simulink model "lego_selfbalance_students"  (R2014a)
settings: Solver=ode3  SolverMode=SingleTasking  StartTime=0.0  StopTime=inf  RelTol=1e-3
values from neighbouring files (symbols this model uses):
  A1 = [ ... (first row only)    [lego_selfbalance_parameters.m]
  A2 = [ ... (first row only)    [lego_selfbalance_parameters.m]
  a_b = 0.8    [lego_selfbalance_parameters.m]
  a_d = 0.8    [lego_selfbalance_parameters.m]
  a_gc = 0.8    [lego_selfbalance_parameters.m]
  a_gd = 0.999    [lego_selfbalance_parameters.m]
  a_r = 0.996    [lego_selfbalance_parameters.m]
  B1 = [ ... (first row only)    [lego_selfbalance_parameters.m]
  B2 = [ ... (first row only)    [lego_selfbalance_parameters.m]
  BATTERY = 8000    [lego_selfbalance_parameters.m]
  C1 = eye(4)    [lego_selfbalance_parameters.m]
  C2 = eye(2)    [lego_selfbalance_parameters.m]
  D = 0.04    [lego_selfbalance_parameters.m]
  D1 = zeros(4, 2)    [lego_selfbalance_parameters.m]
  D2 = zeros(2)    [lego_selfbalance_parameters.m]
  GYRO0 = 600    [lego_selfbalance_parameters.m]
  k_sync = 0.35    [lego_selfbalance_parameters.m]
  pwm_gain = 1    [lego_selfbalance_parameters.m]
  pwm_offset = 0    [lego_selfbalance_parameters.m]
  R = 0.04    [lego_selfbalance_parameters.m]
  START_POS = [100, 100]    [lego_selfbalance_parameters.m]
  time_start = 4000    [lego_selfbalance_parameters.m]
  TS = 0.001    [lego_selfbalance_parameters.m]
  ts1 = 0.004    [lego_selfbalance_parameters.m]
  W = 0.14    [lego_selfbalance_parameters.m]
  X1IV = [ ... (first row only)    [lego_selfbalance_parameters.m]
  X2IV = [ ... (first row only)    [lego_selfbalance_parameters.m]
undefined symbols (not defined in the file or in its folder): DiscIntNeverNeededParam
libraries: legonxtlib x8, simulink x3
PreSaveFcn:
  | set_param(gcs, 'Location',[35 56 895 605])
settings Model: FPTRunName=Active  SimulationMode=external  ExtModeTrigDuration=2  Creator=The MathWorks Inc.  LastModifiedBy=Dan
settings DataIOCC: SignalLoggingSaveFormat=ModelDataLogs
settings OptimizationCC: ExpressionDepthLimit=2147483647  OptimizeModelRefInitCode=on  LifeSpan=Inf
settings DebuggingCC: UnderspecifiedInitializationDetection=Classic  SolverPrmCheckMsg=none  FcnCallInpInsideContextMsg=EnableAllAsWarning  StateNameClashWarn=warning
settings HardwareCC: ProdLargestAtomicInteger=Long  ProdLargestAtomicFloat=Float  ProdEndianess=LittleEndian  ProdHWDeviceType=ARM Compatible->ARM 7
settings RTWCC: SystemTargetFile=realtime.tlc  GenerateMakefile=off  TemplateMakefile=realtime.tmf  Description=Run on Target Hardware  RTWVerbose=off  ProcessScript=realtime_make_rtw_hook
settings CodeAppCC: CustomSymbolStrType=$N$R$M  InternalIdentifier=Classic
settings STFCustomTargetCC: TargetLibSuffix=.a  GenerateSampleERTMain=on  ConcurrentExecutionCompliant=off  GeneratePreprocessorConditionals=Use local settings  ERTCustomFileBanners=on  SupportNonInlinedSFcns=off  SupportVariableSizeSignals=on  MATLABClassNameForMDSCustomization=Simulink.SoftwareTarget.ERTCustomization  GRTInterface=off  SystemTargetFile=realtime.tlc
settings ERTTargetCC: CombineOutputUpdateFcns=off  SupportContinuousTime=on  SupportVariableSizeSignals=on  ExtMode=on  ExtModeTransport=2  ExtModeMexArgs=0 13 9600 30  ERTSrcFileBannerTemplate=realtime_code_template.cgt  ERTHdrFileBannerTemplate=realtime_code_template.cgt  ERTDataSrcFileTemplate=realtime_code_template.cgt  ERTDataHdrFileTemplate=realtime_code_template.cgt  ERTCustomFileTemplate=realtime_file_process.tlc

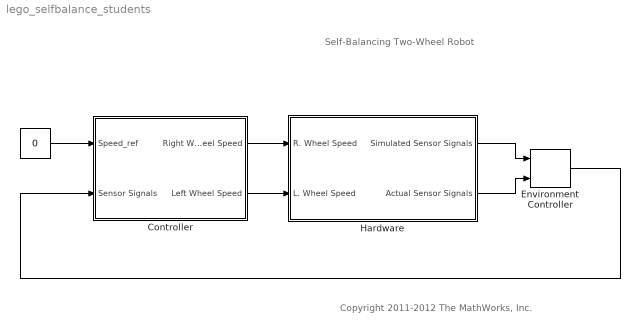
== system lego_selfbalance_students ==
  note: Copyright 2011-2012 The MathWorks, Inc.
  note: Self-Balancing Two-Wheel Robot
  "      " : Constant  Value=0  OutDataTypeStr=single  SampleTime=4*TS
  Controller : Subsystem  TreatAsAtomicUnit=on
  Environment Controller : simulink/Signal Routing/Environment Controller
  Hardware : Subsystem  VariantControl=DoSim
  wires:
  Environment Controller/1 -> Controller/2(Sensor Signals)
  Controller/1(Right Wheel Speed) -> Hardware/1(R. Wheel Speed)
  Controller/2(Left Wheel Speed) -> Hardware/2(L. Wheel Speed)
  Hardware/1(Simulated Sensor Signals) -> Environment Controller/1
  Hardware/2(Actual Sensor Signals) -> Environment Controller/2
  "      "/1 -> Controller/1(Speed_ref)

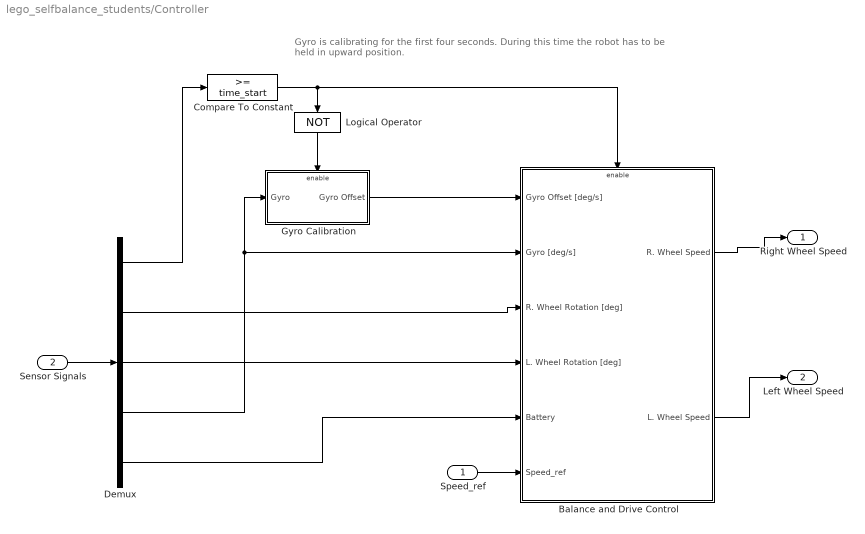
== system lego_selfbalance_students/Controller ==
  note: Gyro is calibrating for the first four seconds.
      | During this time the robot has to be held in upward position.
  Speed_ref : Inport
  Sensor Signals : Inport  Port=2
  Balance and Drive Control : Subsystem
  Compare To Constant : simulink/Logic and Bit Operations/Compare To Constant  relop=>=  const=time_start  OutDataTypeStr=boolean
  Demux : Demux  Outputs=5
  Gyro Calibration : Subsystem  TreatAsAtomicUnit=on
  Logical Operator : Logic  Operator=NOT  AllPortsSameDT=off  OutDataTypeStr=boolean
  Right Wheel Speed : Outport
  Left Wheel Speed : Outport  Port=2
  wires:
  Compare To Constant/1 -> Logical Operator/1, Balance and Drive Control/Enable
  Gyro Calibration/1(Gyro Offset) -> Balance and Drive Control/1(Gyro Offset [deg/s])
  Logical Operator/1 -> Gyro Calibration/Enable
  Sensor Signals/1 -> Demux/1
  Speed_ref/1 -> Balance and Drive Control/6(Speed_ref)
  Demux/3 -> Balance and Drive Control/4(L. Wheel Rotation [deg])
  Demux/2 -> Balance and Drive Control/3(R. Wheel Rotation [deg])
  Demux/1 -> Compare To Constant/1
  Balance and Drive Control/1(R. Wheel Speed) -> Right Wheel Speed/1
  Balance and Drive Control/2(L. Wheel Speed) -> Left Wheel Speed/1
  Demux/4 -> Gyro Calibration/1(Gyro), Balance and Drive Control/2(Gyro [deg/s])
  Demux/5 -> Balance and Drive Control/5(Battery)

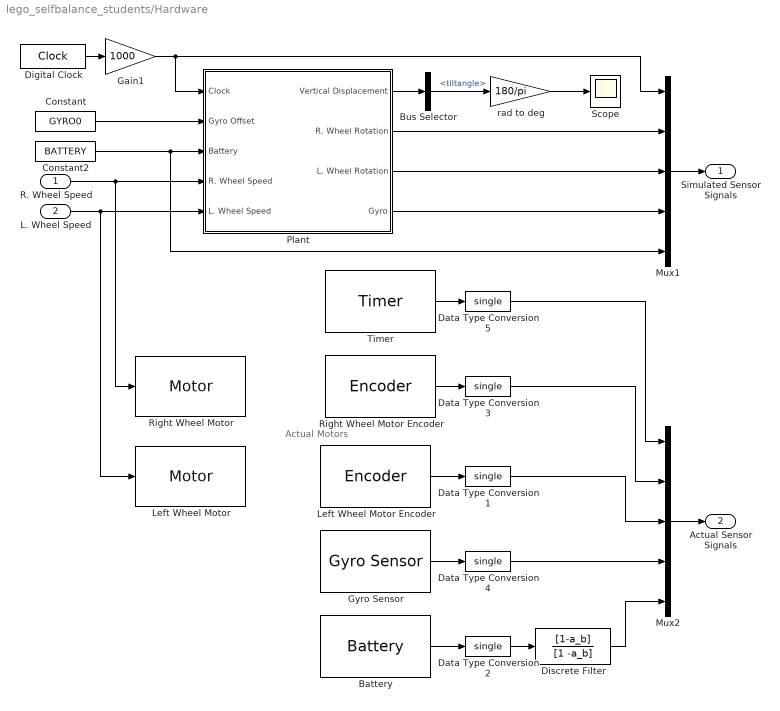
== system lego_selfbalance_students/Hardware ==
  note: Actual
      | Motors
  R. Wheel Speed : Inport
  L. Wheel Speed : Inport  Port=2
  Battery : legonxtlib/Battery  sampleTime=ts1
  Bus Selector : BusSelector  OutputSignals=tiltangle
  Constant : Constant  Value=GYRO0  OutDataTypeStr=single
  Constant2 : Constant  Value=BATTERY  OutDataTypeStr=single
  Data Type Conversion{1..5} (5 alike) : DataTypeConversion  OutDataTypeStr=single  RndMeth=Simplest
  Digital Clock : DigitalClock  SampleTime=4*TS
  Discrete Filter : DiscreteFilter  Numerator=[1-a_b]  Denominator=[1 -a_b]
  Gain1 : Gain  Gain=1000  OutDataTypeStr=single  ParamDataTypeStr=Inherit: Same as input
  Gyro Sensor : legonxtlib/Gyro Sensor  portNumber=4  outputMode=Raw A/D (0 - 1023)  offset=600  sampleTime=ts1
  Left Wheel Motor : legonxtlib/Motor  sportNumber=C  sstopAction=Brake
  Left Wheel Motor Encoder : legonxtlib/Encoder  portNumber=C  opMode=No reset  sampleTime=ts1
  Mux1 : Mux  Inputs=5
  Mux2 : Mux  Inputs=5
  Plant : Subsystem
  Right Wheel Motor : legonxtlib/Motor  sportNumber=B  sstopAction=Brake
  Right Wheel Motor Encoder : legonxtlib/Encoder  portNumber=B  opMode=No reset  sampleTime=ts1
  Scope : Scope
      settings: YMin=-8  YMax=8
  Timer : legonxtlib/Timer  sampleTime=ts1
  rad to deg : Gain  Gain=180/pi
  Simulated Sensor Signals : Outport
  Actual Sensor Signals : Outport  Port=2
  wires:
  Data Type Conversion5/1 -> Mux2/1
  Timer/1 -> Data Type Conversion5/1
  Data Type Conversion4/1 -> Mux2/4
  Data Type Conversion1/1 -> Mux2/3
  Data Type Conversion3/1 -> Mux2/2
  Mux2/1 -> Actual Sensor Signals/1
  Left Wheel Motor Encoder/1 -> Data Type Conversion1/1
  Right Wheel Motor Encoder/1 -> Data Type Conversion3/1
  Battery/1 -> Data Type Conversion2/1
  Data Type Conversion2/1 -> Discrete Filter/1
  Discrete Filter/1 -> Mux2/5
  Gyro Sensor/1 -> Data Type Conversion4/1
  L. Wheel Speed/1 -> Plant/5(L. Wheel Speed), Left Wheel Motor/1
  Mux1/1 -> Simulated Sensor Signals/1
  Plant/3(L. Wheel Rotation) -> Mux1/3
  R. Wheel Speed/1 -> Plant/4(R. Wheel Speed), Right Wheel Motor/1
  Constant2/1 -> Mux1/5, Plant/3(Battery)
  Plant/2(R. Wheel Rotation) -> Mux1/2
  Plant/4(Gyro) -> Mux1/4
  Digital Clock/1 -> Gain1/1
  Gain1/1 -> Mux1/1, Plant/1(Clock)
  rad to deg/1 -> Scope/1
  Plant/1(Vertical Displacement) -> Bus Selector/1
  Bus Selector/1 -> rad to deg/1  "<tiltangle>"
  Constant/1 -> Plant/2(Gyro Offset)

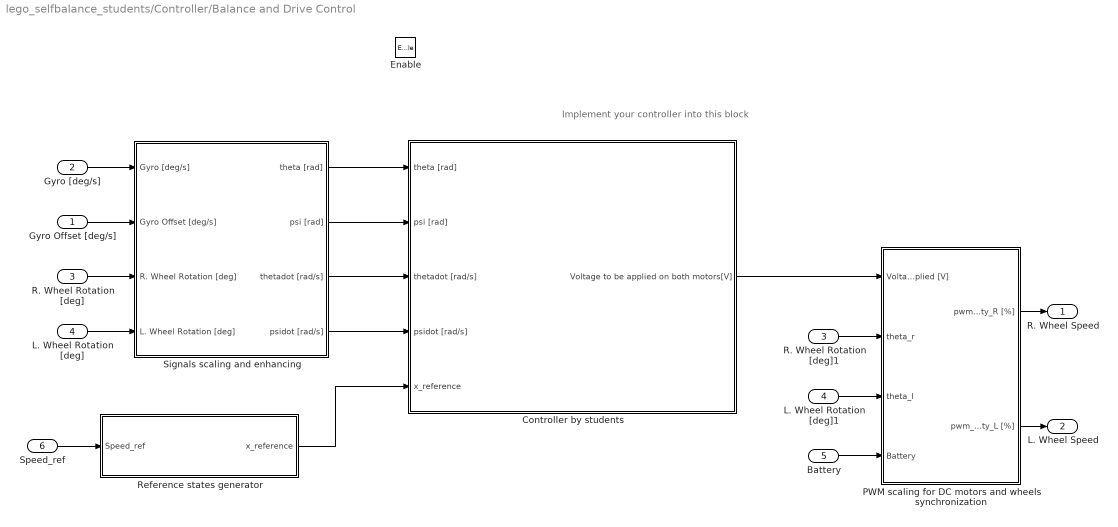
== system lego_selfbalance_students/Controller/Balance and Drive Control ==
  note: Implement your controller into this block
  Gyro Offset [deg/s] : Inport
  Gyro [deg/s] : Inport  Port=2
  R. Wheel Rotation [deg] : Inport  Port=3
  L. Wheel Rotation [deg] : Inport  Port=4
  Battery : Inport  Port=5
  Speed_ref : Inport  Port=6
  Enable : EnablePort
  "Controller by students " : Subsystem
  L. Wheel Rotation [deg]1 : InportShadow  Port=4
  PWM scaling for DC motors and wheels synchronization : Subsystem
  R. Wheel Rotation [deg]1 : InportShadow  Port=3
  Reference states generator : Subsystem
  Signals scaling and enhancing : Subsystem
  R. Wheel Speed : Outport
  L. Wheel Speed : Outport  Port=2
  wires:
  L. Wheel Rotation [deg]/1 -> Signals scaling and enhancing/4(L. Wheel Rotation [deg])
  Battery/1 -> PWM scaling for DC motors and wheels synchronization/4(Battery)
  R. Wheel Rotation [deg]/1 -> Signals scaling and enhancing/3(R. Wheel Rotation [deg])
  Gyro [deg/s]/1 -> Signals scaling and enhancing/1(Gyro [deg/s])
  Gyro Offset [deg/s]/1 -> Signals scaling and enhancing/2(Gyro Offset [deg/s])
  PWM scaling for DC motors and wheels synchronization/2(pwm_duty_L [%]) -> L. Wheel Speed/1
  PWM scaling for DC motors and wheels synchronization/1(pwm_duty_R [%]) -> R. Wheel Speed/1
  Signals scaling and enhancing/4(psidot [rad/s]) -> "Controller by students "/4(psidot [rad/s])
  "Controller by students "/1(Voltage to be applied on both motors[V]) -> PWM scaling for DC motors and wheels synchronization/1(Voltage to be applied [V])
  Speed_ref/1 -> Reference states generator/1(Speed_ref)
  Reference states generator/1(x_reference) -> "Controller by students "/5(x_reference)
  R. Wheel Rotation [deg]1/1 -> PWM scaling for DC motors and wheels synchronization/2(theta_r)
  L. Wheel Rotation [deg]1/1 -> PWM scaling for DC motors and wheels synchronization/3(theta_l)
  Signals scaling and enhancing/1(theta [rad]) -> "Controller by students "/1(theta [rad])
  Signals scaling and enhancing/2(psi [rad]) -> "Controller by students "/2(psi [rad])
  Signals scaling and enhancing/3(thetadot [rad/s]) -> "Controller by students "/3(thetadot [rad/s])

== system lego_selfbalance_students/Controller/Gyro Calibration ==
  note: Calculate gyro offset
  Gyro : Inport
  Enable : EnablePort
  Constant : Constant  Value=440  OutDataTypeStr=uint32  SampleTime=0.2
  Gain2 : Gain  Gain=1-a_gc  OutDataTypeStr=Inherit: Same as input  ParamDataTypeStr=Inherit: Same as input
  Gain3 : Gain  Gain=a_gc  OutDataTypeStr=Inherit: Same as input  ParamDataTypeStr=Inherit: Same as input
  Speaker : legonxtlib/Speaker  sinputMode=Frequency only  sspeakerFreq=100  sspeakerVolume=10  sspeakerDuration=100
  Sum1 : Sum  Inputs=|++  OutDataTypeStr=Inherit: Same as first input
  Unit Delay : UnitDelay  SampleTime=-1
  Gyro Offset : Outport
  wires:
  Gain3/1 -> Sum1/2
  Unit Delay/1 -> Gain3/1
  Sum1/1 -> Unit Delay/1, Gyro Offset/1
  Gain2/1 -> Sum1/1
  Gyro/1 -> Gain2/1
  Constant/1 -> Speaker/1

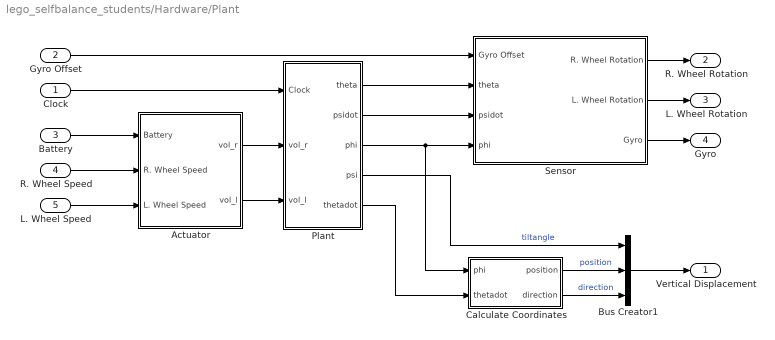
== system lego_selfbalance_students/Hardware/Plant ==
  Clock : Inport
  Gyro Offset : Inport  Port=2
  Battery : Inport  Port=3
  R. Wheel Speed : Inport  Port=4
  L. Wheel Speed : Inport  Port=5
  Actuator : Subsystem
  Bus Creator1 : BusCreator  Inputs=3
  Calculate Coordinates : Subsystem
  Plant : Subsystem
  Sensor : Subsystem
  Vertical Displacement : Outport
  R. Wheel Rotation : Outport  Port=2
  L. Wheel Rotation : Outport  Port=3
  Gyro : Outport  Port=4
  wires:
  Clock/1 -> Plant/1(Clock)
  Plant/4(psi) -> Bus Creator1/1  "tiltangle"
  Bus Creator1/1 -> Vertical Displacement/1
  Calculate Coordinates/2(direction) -> Bus Creator1/3  "direction"
  Calculate Coordinates/1(position) -> Bus Creator1/2  "position"
  Plant/3(phi) -> Calculate Coordinates/1(phi), Sensor/4(phi)
  L. Wheel Speed/1 -> Actuator/3(L. Wheel Speed)
  Plant/5(thetadot) -> Calculate Coordinates/2(thetadot)
  Sensor/3(Gyro) -> Gyro/1
  R. Wheel Speed/1 -> Actuator/2(R. Wheel Speed)
  Sensor/2(L. Wheel Rotation) -> L. Wheel Rotation/1
  Sensor/1(R. Wheel Rotation) -> R. Wheel Rotation/1
  Gyro Offset/1 -> Sensor/1(Gyro Offset)
  Battery/1 -> Actuator/1(Battery)
  Plant/1(theta) -> Sensor/2(theta)
  Plant/2(psidot) -> Sensor/3(psidot)
  Actuator/2(vol_l) -> Plant/3(vol_l)
  Actuator/1(vol_r) -> Plant/2(vol_r)

== system lego_selfbalance_students/Controller/Balance and Drive Control/Controller by students  ==
  note: Your controller should be implemented here
  theta [rad] : Inport
  psi [rad] : Inport  Port=2
  thetadot [rad/s] : Inport  Port=3
  psidot [rad/s] : Inport  Port=4
  x_reference : Inport  Port=5
  Measured outputs : Scope
      settings: SaveName=ScopeData2
  Mux1 : Mux
  Voltage to be applied on both motors[V] : Outport
  wires:
  psi [rad]/1 -> Mux1/2
  thetadot [rad/s]/1 -> Mux1/3
  psidot [rad/s]/1 -> Mux1/4
  Mux1/1 -> Measured outputs/1
  theta [rad]/1 -> Mux1/1

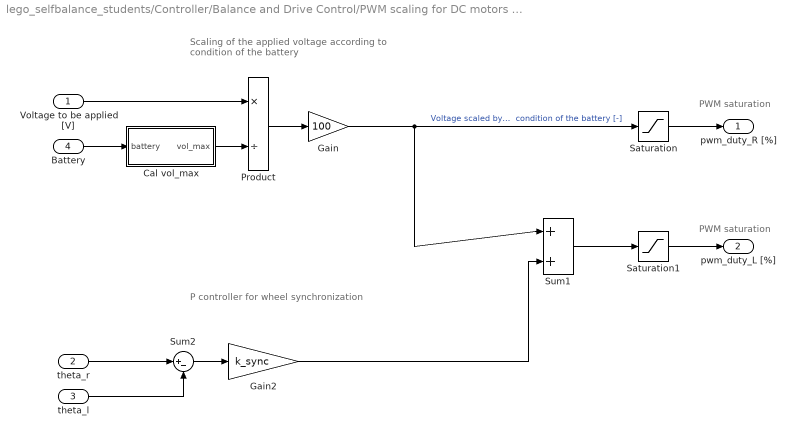
== system lego_selfbalance_students/Controller/Balance and Drive Control/PWM scaling for DC motors and wheels synchronization ==
  note: PWM saturation
  note: P controller for wheel synchronization
  note: Scaling of the applied voltage
      | according to condition of the battery
  note: PWM saturation
  Voltage to be applied [V] : Inport
  theta_r : Inport  Port=2
  theta_l : Inport  Port=3
  Battery : Inport  Port=4
  Cal vol_max : Subsystem
  Gain : Gain  Gain=100  OutDataTypeStr=Inherit: Same as input  ParamDataTypeStr=Inherit: Same as input
  Gain2 : Gain  Gain=k_sync  OutDataTypeStr=Inherit: Same as input  ParamDataTypeStr=Inherit: Same as input
  Product : Product  Inputs=*/  RndMeth=Simplest  OutDataTypeStr=Inherit: Same as first input
  Saturation : Saturate  UpperLimit=100  LowerLimit=-100
      settings: AttributesFormatString=max = %<UpperLimit>\nmin = %<LowerLimit>
  Saturation1 : Saturate  UpperLimit=100  LowerLimit=-100
      settings: AttributesFormatString=max = %<UpperLimit>\nmin = %<LowerLimit>
  Sum1 : Sum  Inputs=|++  OutDataTypeStr=Inherit: Same as first input
  Sum2 : Sum  Inputs=|+-  OutDataTypeStr=Inherit: Same as first input
  pwm_duty_R [%] : Outport
  pwm_duty_L [%] : Outport  Port=2
  wires:
  Cal vol_max/1(vol_max) -> Product/2
  Battery/1 -> Cal vol_max/1(battery)
  Product/1 -> Gain/1
  Voltage to be applied [V]/1 -> Product/1
  Gain/1 -> Sum1/1, Saturation/1  "Voltage scaled by  condition of the battery [-]"
  Saturation/1 -> pwm_duty_R [%]/1
  Saturation1/1 -> pwm_duty_L [%]/1
  theta_r/1 -> Sum2/1
  Sum1/1 -> Saturation1/1
  Sum2/1 -> Gain2/1
  theta_l/1 -> Sum2/2
  Gain2/1 -> Sum1/2

== system lego_selfbalance_students/Controller/Balance and Drive Control/Reference states generator ==
  Speed_ref : Inport
  Constant2 : Constant  Value=0  VectorParams1D=off  OutDataTypeStr=single
  Constant3 : Constant  Value=0  VectorParams1D=off  OutDataTypeStr=single
  Discrete Integrator (Forward Euler)1 : Subsystem
  Filter : Subsystem
  Mux : Mux
  x_reference : Outport
  wires:
  Discrete Integrator (Forward Euler)1/1(out) -> Mux/1  "theta_ref"
  Constant2/1 -> Mux/2  "psi_ref"
  Speed_ref/1 -> Filter/1(in)
  Constant3/1 -> Mux/4  "psidot_ref"
  Mux/1 -> x_reference/1
  Filter/1(out) -> Mux/3, Discrete Integrator (Forward Euler)1/1(in)  "thetadot_ref"

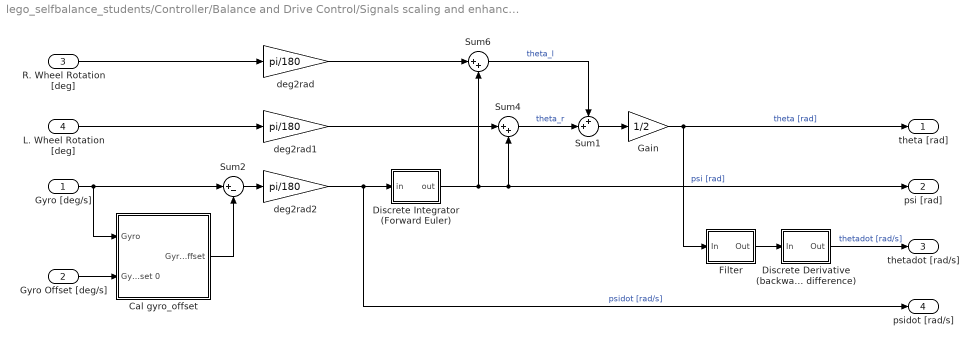
== system lego_selfbalance_students/Controller/Balance and Drive Control/Signals scaling and enhancing ==
  Gyro [deg/s] : Inport
  Gyro Offset [deg/s] : Inport  Port=2
  R. Wheel Rotation [deg] : Inport  Port=3
  L. Wheel Rotation [deg] : Inport  Port=4
  Cal gyro_offset : Subsystem
  Discrete Derivative (backward difference) : Subsystem
  Discrete Integrator (Forward Euler) : Subsystem
  Filter : Subsystem
  Gain : Gain  Gain=1/2  OutDataTypeStr=Inherit: Same as input  ParamDataTypeStr=Inherit: Same as input
  Sum1 : Sum  Inputs=++|  OutDataTypeStr=Inherit: Same as first input
  Sum2 : Sum  Inputs=|+-  OutDataTypeStr=Inherit: Same as first input
  Sum4 : Sum  Inputs=|++  OutDataTypeStr=Inherit: Same as first input
  Sum6 : Sum  Inputs=|++  OutDataTypeStr=Inherit: Same as first input
  deg2rad : Gain  Gain=pi/180  OutDataTypeStr=Inherit: Same as input  ParamDataTypeStr=Inherit: Same as input
  deg2rad1 : Gain  Gain=pi/180  OutDataTypeStr=Inherit: Same as input  ParamDataTypeStr=Inherit: Same as input
  deg2rad2 : Gain  Gain=pi/180  OutDataTypeStr=Inherit: Same as input  ParamDataTypeStr=Inherit: Same as input
  theta [rad] : Outport
  psi [rad] : Outport  Port=2
  thetadot [rad/s] : Outport  Port=3
  psidot [rad/s] : Outport  Port=4
  wires:
  Gain/1 -> theta [rad]/1, Filter/1(In)  "theta [rad]"
  Filter/1(Out) -> Discrete Derivative (backward difference)/1(In)
  deg2rad2/1 -> psidot [rad/s]/1, Discrete Integrator (Forward Euler)/1(in)  "psidot [rad/s]"
  Sum1/1 -> Gain/1
  Sum4/1 -> Sum1/2  "theta_r"
  Sum6/1 -> Sum1/1  "theta_l"
  Discrete Derivative (backward difference)/1(Out) -> thetadot [rad/s]/1  "thetadot [rad/s]"
  L. Wheel Rotation [deg]/1 -> deg2rad1/1
  R. Wheel Rotation [deg]/1 -> deg2rad/1
  deg2rad/1 -> Sum6/1
  Discrete Integrator (Forward Euler)/1(out) -> Sum6/2, psi [rad]/1, Sum4/2  "psi [rad]"
  deg2rad1/1 -> Sum4/1
  Gyro [deg/s]/1 -> Sum2/1, Cal gyro_offset/1(Gyro)
  Sum2/1 -> deg2rad2/1
  Cal gyro_offset/1(Gyro Offset) -> Sum2/2
  Gyro Offset [deg/s]/1 -> Cal gyro_offset/2(Gyro Offset 0)

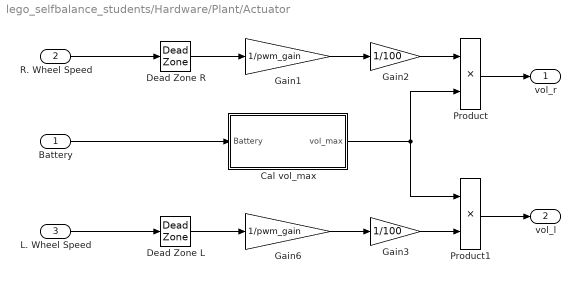
== system lego_selfbalance_students/Hardware/Plant/Actuator ==
  Battery : Inport
  R. Wheel Speed : Inport  Port=2
  L. Wheel Speed : Inport  Port=3
  Cal vol_max : Subsystem
  Dead Zone L : DeadZone  LowerValue=-pwm_offset  UpperValue=pwm_offset  SaturateOnIntegerOverflow=on
      settings: AttributesFormatString=start=%<LowerValue>\nend=%<UpperValue>
  Dead Zone R : DeadZone  LowerValue=-pwm_offset  UpperValue=pwm_offset  SaturateOnIntegerOverflow=on
      settings: AttributesFormatString=start=%<LowerValue>\nend=%<UpperValue>
  Gain1 : Gain  Gain=1/pwm_gain  OutDataTypeStr=Inherit: Same as input  ParamDataTypeStr=Inherit: Same as input
  Gain2 : Gain  Gain=1/100  OutDataTypeStr=Inherit: Same as input  ParamDataTypeStr=Inherit: Same as input
  Gain3 : Gain  Gain=1/100  OutDataTypeStr=Inherit: Same as input  ParamDataTypeStr=Inherit: Same as input
  Gain6 : Gain  Gain=1/pwm_gain  OutDataTypeStr=Inherit: Same as input  ParamDataTypeStr=Inherit: Same as input
  Product : Product  RndMeth=Simplest
  Product1 : Product  RndMeth=Simplest
  vol_r : Outport
  vol_l : Outport  Port=2
  wires:
  Battery/1 -> Cal vol_max/1(Battery)
  Cal vol_max/1(vol_max) -> Product1/1, Product/2
  Dead Zone R/1 -> Gain1/1
  Product1/1 -> vol_l/1
  Gain3/1 -> Product1/2
  Product/1 -> vol_r/1
  Gain2/1 -> Product/1
  Gain6/1 -> Gain3/1
  Gain1/1 -> Gain2/1
  L. Wheel Speed/1 -> Dead Zone L/1
  R. Wheel Speed/1 -> Dead Zone R/1
  Dead Zone L/1 -> Gain6/1

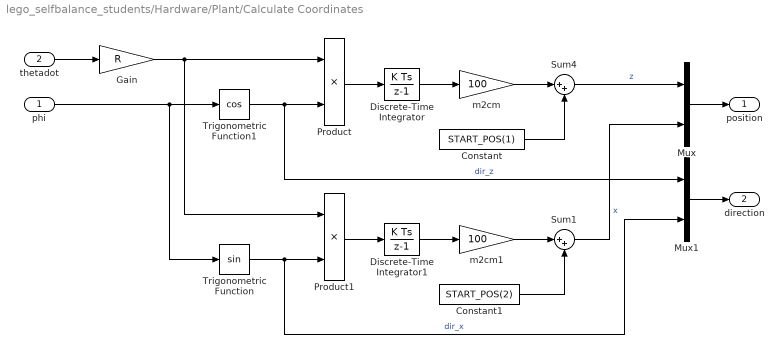
== system lego_selfbalance_students/Hardware/Plant/Calculate Coordinates ==
  phi : Inport
  thetadot : Inport  Port=2
  Constant : Constant  Value=START_POS(1)  OutDataTypeStr=double
      settings: AttributesFormatString=DataType = %<OutDataTypeStr>
  Constant1 : Constant  Value=START_POS(2)  OutDataTypeStr=double
      settings: AttributesFormatString=DataType = %<OutDataTypeStr>
  Discrete-Time Integrator : DiscreteIntegrator  SampleTime=4*TS  ICPrevOutput=DiscIntNeverNeededParam  ICPrevScaledInput=DiscIntNeverNeededParam
  Discrete-Time Integrator1 : DiscreteIntegrator  SampleTime=4*TS  ICPrevOutput=DiscIntNeverNeededParam  ICPrevScaledInput=DiscIntNeverNeededParam
  Gain : Gain  Gain=R
  Mux : Mux  Inputs=2
  Mux1 : Mux  Inputs=2
  Product : Product  OutDataTypeStr=double  RndMeth=Simplest
  Product1 : Product  OutDataTypeStr=double  RndMeth=Simplest
  Sum1 : Sum  Inputs=|++
  Sum4 : Sum  Inputs=|++
  Trigonometric Function : Trigonometry
  Trigonometric Function1 : Trigonometry  Operator=cos
  m2cm : Gain  Gain=100
  m2cm1 : Gain  Gain=100
  position : Outport
  direction : Outport  Port=2
  wires:
  Mux1/1 -> direction/1
  Mux/1 -> position/1
  Sum1/1 -> Mux/2  "x"
  Constant1/1 -> Sum1/2
  m2cm1/1 -> Sum1/1
  Constant/1 -> Sum4/2
  Sum4/1 -> Mux/1  "z"
  m2cm/1 -> Sum4/1
  Gain/1 -> Product/1, Product1/1
  Discrete-Time Integrator1/1 -> m2cm1/1
  Discrete-Time Integrator/1 -> m2cm/1
  phi/1 -> Trigonometric Function/1, Trigonometric Function1/1
  thetadot/1 -> Gain/1
  Trigonometric Function1/1 -> Mux1/1, Product/2  "dir_z"
  Product/1 -> Discrete-Time Integrator/1
  Trigonometric Function/1 -> Mux1/2, Product1/2  "dir_x"
  Product1/1 -> Discrete-Time Integrator1/1

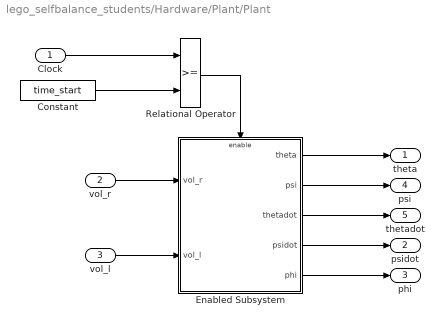
== system lego_selfbalance_students/Hardware/Plant/Plant ==
  Clock : Inport
  vol_r : Inport  Port=2
  vol_l : Inport  Port=3
  Constant : Constant  Value=time_start  OutDataTypeStr=single
  Enabled Subsystem : Subsystem  TreatAsAtomicUnit=on
      settings: MinAlgLoopOccurrences=on
  Relational Operator : RelationalOperator  OutDataTypeStr=boolean
  theta : Outport
  psidot : Outport  Port=2
  phi : Outport  Port=3
  psi : Outport  Port=4
  thetadot : Outport  Port=5
  wires:
  Enabled Subsystem/4(psidot) -> psidot/1
  Enabled Subsystem/5(phi) -> phi/1
  Enabled Subsystem/2(psi) -> psi/1
  Enabled Subsystem/3(thetadot) -> thetadot/1
  Enabled Subsystem/1(theta) -> theta/1
  Constant/1 -> Relational Operator/2
  Clock/1 -> Relational Operator/1
  Relational Operator/1 -> Enabled Subsystem/Enable
  vol_l/1 -> Enabled Subsystem/2(vol_l)
  vol_r/1 -> Enabled Subsystem/1(vol_r)

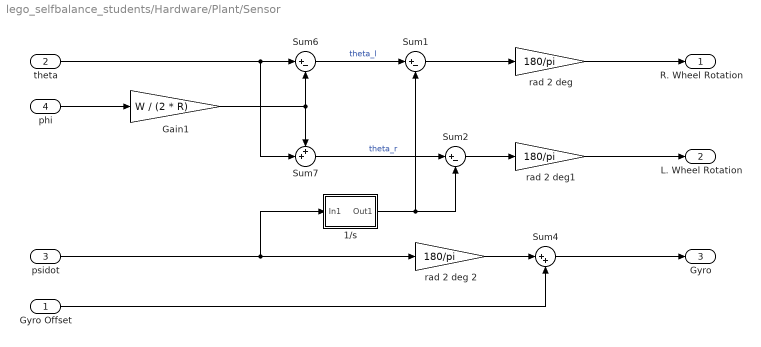
== system lego_selfbalance_students/Hardware/Plant/Sensor ==
  Gyro Offset : Inport
  theta : Inport  Port=2
  psidot : Inport  Port=3
  phi : Inport  Port=4
  1/s : Subsystem
  Gain1 : Gain  Gain=W / (2 * R)
  Sum1 : Sum  Inputs=|+-
  Sum2 : Sum  Inputs=|+-
  Sum4 : Sum  Inputs=|++
  Sum6 : Sum  Inputs=|+-
  Sum7 : Sum  Inputs=++|
  rad 2 deg : Gain  Gain=180/pi  OutDataTypeStr=single
  rad 2 deg 2 : Gain  Gain=180/pi
  rad 2 deg1 : Gain  Gain=180/pi  OutDataTypeStr=single
  R. Wheel Rotation : Outport
  L. Wheel Rotation : Outport  Port=2
  Gyro : Outport  Port=3
  wires:
  1/s/1(Out1) -> Sum1/2, Sum2/2
  Sum6/1 -> Sum1/1  "theta_l"
  rad 2 deg1/1 -> L. Wheel Rotation/1
  rad 2 deg/1 -> R. Wheel Rotation/1
  Sum2/1 -> rad 2 deg1/1
  psidot/1 -> 1/s/1(In1), rad 2 deg 2/1
  Sum1/1 -> rad 2 deg/1
  Gain1/1 -> Sum6/2, Sum7/1
  phi/1 -> Gain1/1
  theta/1 -> Sum6/1, Sum7/2
  rad 2 deg 2/1 -> Sum4/1
  Sum7/1 -> Sum2/1  "theta_r"
  Gyro Offset/1 -> Sum4/2
  Sum4/1 -> Gyro/1

== system lego_selfbalance_students/Controller/Balance and Drive Control/PWM scaling for DC motors and wheels synchronization/Cal vol_max ==
  battery : Inport
  Constant : Constant  Value=0.625  OutDataTypeStr=single
      settings: AttributesFormatString=DataType = %<OutDataTypeStr>
  Gain3 : Gain  Gain=0.001089  OutDataTypeStr=Inherit: Same as input  ParamDataTypeStr=Inherit: Same as input
  Sum2 : Sum  Inputs=|+-  OutDataTypeStr=Inherit: Same as first input
  vol_max : Outport
  wires:
  Gain3/1 -> Sum2/1
  Sum2/1 -> vol_max/1
  Constant/1 -> Sum2/2
  battery/1 -> Gain3/1

== system lego_selfbalance_students/Controller/Balance and Drive Control/Reference states generator/Discrete Integrator (Forward Euler)1 ==
  in : Inport
  Gain : Gain  Gain=ts1  OutDataTypeStr=Inherit: Same as input  ParamDataTypeStr=Inherit: Same as input
  Sum : Sum  Inputs=|++  OutDataTypeStr=Inherit: Same as first input
  Unit Delay : UnitDelay  SampleTime=-1
  out : Outport
  wires:
  in/1 -> Gain/1
  Sum/1 -> Unit Delay/1
  Gain/1 -> Sum/1
  Unit Delay/1 -> out/1, Sum/2

== system lego_selfbalance_students/Controller/Balance and Drive Control/Reference states generator/Filter ==
  note: Filter Function:
      |               1-a_r
      |          ----------------
      |          1-a_r*z^(-1)
  in : Inport
  Gain2 : Gain  Gain=a_r  OutDataTypeStr=Inherit: Same as input  ParamDataTypeStr=Inherit: Same as input
  Gain3 : Gain  Gain=1-a_r  OutDataTypeStr=Inherit: Same as input  ParamDataTypeStr=Inherit: Same as input
  Sum : Sum  Inputs=|++  OutDataTypeStr=Inherit: Same as first input
  Unit Delay : UnitDelay  SampleTime=-1
  out : Outport
  wires:
  in/1 -> Gain3/1
  Gain3/1 -> Sum/1
  Gain2/1 -> Sum/2
  Unit Delay/1 -> Gain2/1
  Sum/1 -> out/1, Unit Delay/1

== system lego_selfbalance_students/Controller/Balance and Drive Control/Signals scaling and enhancing/Cal gyro_offset ==
  Gyro : Inport
  Gyro Offset 0 : Inport  Port=2
  Gain1 : Gain  Gain=1-a_gd  OutDataTypeStr=Inherit: Same as input  ParamDataTypeStr=Inherit: Same as input
  Gain4 : Gain  Gain=a_gd  OutDataTypeStr=Inherit: Same as input  ParamDataTypeStr=Inherit: Same as input
  Sum2 : Sum  Inputs=|++  OutDataTypeStr=Inherit: Same as first input
  Unit Delay External IC : simulink/Additional Math & Discrete/Additional Discrete/Unit Delay External IC  tsamp=-1
  Gyro Offset : Outport
  wires:
  Gyro/1 -> Gain1/1
  Gyro Offset 0/1 -> Unit Delay External IC/2
  Gain1/1 -> Sum2/1
  Sum2/1 -> Gyro Offset/1, Unit Delay External IC/1
  Unit Delay External IC/1 -> Gain4/1
  Gain4/1 -> Sum2/2

== system lego_selfbalance_students/Controller/Balance and Drive Control/Signals scaling and enhancing/Discrete Derivative (backward difference) ==
  In : Inport
  Gain : Gain  Gain=1/ts1  OutDataTypeStr=Inherit: Same as input  ParamDataTypeStr=Inherit: Same as input
  Sum : Sum  Inputs=|+-  OutDataTypeStr=Inherit: Same as first input
  Unit Delay : UnitDelay  SampleTime=-1
  Out : Outport
  wires:
  Gain/1 -> Out/1
  In/1 -> Sum/1, Unit Delay/1
  Unit Delay/1 -> Sum/2
  Sum/1 -> Gain/1

== system lego_selfbalance_students/Controller/Balance and Drive Control/Signals scaling and enhancing/Discrete Integrator (Forward Euler) ==
  in : Inport
  Gain : Gain  Gain=ts1  OutDataTypeStr=Inherit: Same as input  ParamDataTypeStr=Inherit: Same as input
  Sum : Sum  Inputs=|++  OutDataTypeStr=Inherit: Same as first input
  Unit Delay : UnitDelay  SampleTime=-1
  out : Outport
  wires:
  Unit Delay/1 -> Sum/2, out/1
  Gain/1 -> Sum/1
  Sum/1 -> Unit Delay/1
  in/1 -> Gain/1

== system lego_selfbalance_students/Controller/Balance and Drive Control/Signals scaling and enhancing/Filter ==
  In : Inport
  Gain2 : Gain  Gain=a_d  OutDataTypeStr=Inherit: Same as input  ParamDataTypeStr=Inherit: Same as input
  Gain3 : Gain  Gain=1-a_d  OutDataTypeStr=Inherit: Same as input  ParamDataTypeStr=Inherit: Same as input
  Sum : Sum  Inputs=|++  OutDataTypeStr=Inherit: Same as first input
  Unit Delay : UnitDelay  SampleTime=-1
  Out : Outport
  wires:
  In/1 -> Gain3/1
  Gain3/1 -> Sum/1
  Gain2/1 -> Sum/2
  Unit Delay/1 -> Gain2/1
  Sum/1 -> Out/1, Unit Delay/1

== system lego_selfbalance_students/Hardware/Plant/Actuator/Cal vol_max ==
  note: Calculate maximum DC motor (battery)
      | voltage using an experimental expression
  Battery : Inport
  Constant : Constant  Value=0.625  OutDataTypeStr=single
  Gain3 : Gain  Gain=0.001089  OutDataTypeStr=Inherit: Same as input  ParamDataTypeStr=Inherit: Same as input
  Sum2 : Sum  Inputs=|+-  OutDataTypeStr=Inherit: Same as first input
  vol_max : Outport
  wires:
  Constant/1 -> Sum2/2
  Sum2/1 -> vol_max/1
  Gain3/1 -> Sum2/1
  Battery/1 -> Gain3/1

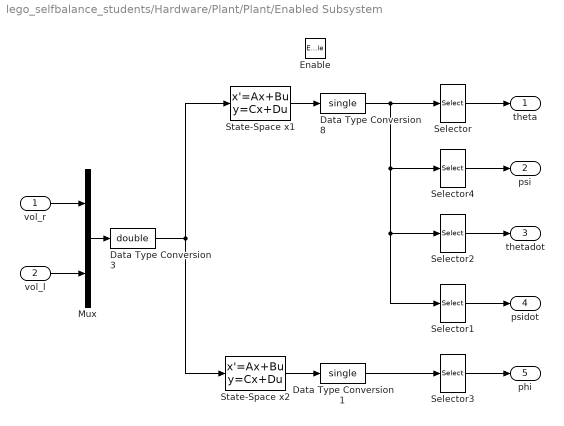
== system lego_selfbalance_students/Hardware/Plant/Plant/Enabled Subsystem ==
  vol_r : Inport
  vol_l : Inport  Port=2
  Enable : EnablePort
  Data Type Conversion1 : DataTypeConversion  OutDataTypeStr=single  RndMeth=Nearest
  Data Type Conversion3 : DataTypeConversion  OutDataTypeStr=double  RndMeth=Nearest
  Data Type Conversion8 : DataTypeConversion  OutDataTypeStr=single  RndMeth=Nearest
  Mux : Mux  Inputs=2
  Selector : Selector  InputPortWidth=4
  Selector1 : Selector  InputPortWidth=4  Indices=4
  Selector2 : Selector  InputPortWidth=4  Indices=3
  Selector3 : Selector  InputPortWidth=2
  Selector4 : Selector  InputPortWidth=4  Indices=2
  State-Space x1 : StateSpace  A=A1  B=B1  C=C1  D=D1  X0=X1IV
  State-Space x2 : StateSpace  A=A2  B=B2  C=C2  D=D2  X0=X2IV
  theta : Outport  InitialOutput=0
  psi : Outport  Port=2  InitialOutput=0
  thetadot : Outport  Port=3  InitialOutput=0
  psidot : Outport  Port=4  InitialOutput=0
  phi : Outport  Port=5  InitialOutput=0
  wires:
  Data Type Conversion1/1 -> Selector3/1
  Data Type Conversion3/1 -> State-Space x1/1, State-Space x2/1
  Data Type Conversion8/1 -> Selector2/1, Selector1/1, Selector4/1, Selector/1
  Selector1/1 -> psidot/1
  Selector/1 -> theta/1
  Selector4/1 -> psi/1
  Selector2/1 -> thetadot/1
  Selector3/1 -> phi/1
  Mux/1 -> Data Type Conversion3/1
  vol_l/1 -> Mux/2
  vol_r/1 -> Mux/1
  State-Space x1/1 -> Data Type Conversion8/1
  State-Space x2/1 -> Data Type Conversion1/1

== system lego_selfbalance_students/Hardware/Plant/Sensor/1//s ==
  In1 : Inport
  Data Type Conversion1 : DataTypeConversion  OutDataTypeStr=double  RndMeth=Nearest
      settings: AttributesFormatString=Round = %<RndMeth>
  Discrete-Time Integrator : DiscreteIntegrator  gainval=1  SampleTime=4*TS  ICPrevOutput=DiscIntNeverNeededParam  ICPrevScaledInput=DiscIntNeverNeededParam
  Out1 : Outport
  wires:
  In1/1 -> Data Type Conversion1/1
  Data Type Conversion1/1 -> Discrete-Time Integrator/1
  Discrete-Time Integrator/1 -> Out1/1
